simulink model "receive"  (R2024b)
settings: Solver=FixedStepAuto  StartTime=0.0  StopTime=10.0  RelTol=1e-3
settings Model: Creator=Amin  LastModifiedBy=Amin
settings OptimizationCC: DefaultParameterBehavior=Inlined  EnhancedBackFolding=on  PassReuseOutputArgsAs=Individual arguments  ZeroExternalMemoryAtStartup=off  ZeroInternalMemoryAtStartup=off  OptimizeBlockOrder=speed  DifferentSizesBufferReuse=on  OptimizationCustomize=off  EfficientTunableParamExpr=on
settings DebuggingCC: ParameterTunabilityLossMsg=error
settings SFSimCC: MATLABDynamicMemAlloc=off
settings RTWCC: Description=Embedded Coder  SystemTargetFile=ert.tlc  GenCodeOnly=on  TemplateMakefile=ert_default_tmf  DataTypeReplacement=CDataTypesFixedWidth  TargetLang=C++
settings CodeAppCC: ForceParamTrailComments=on  IgnoreCustomStorageClasses=off  OperatorAnnotations=on  SimulinkDataObjDesc=on  SFDataObjDesc=on  InsertBlockDesc=on
settings ERTTargetCC: TargetLangStandard=C++11 (ISO)  GenerateSampleERTMain=on  SupportAbsoluteTime=off  CodeInterfacePackaging=C++ class  SupportNonFinite=off  SupportComplex=off  RootIOFormat=Structure reference  ERTCustomFileTemplate=example_file_process.tlc  ERTFilePackagingFormat=Compact  MaxIdInt64=INT64_MAX  MinIdInt64=INT64_MIN  MaxIdUint64=UINT64_MAX  MaxIdInt32=INT32_MAX  MinIdInt32=INT32_MIN  MaxIdUint32=UINT32_MAX  MaxIdInt16=INT16_MAX  MinIdInt16=INT16_MIN  MaxIdUint16=UINT16_MAX  MaxIdInt8=INT8_MAX  MinIdInt8=INT8_MIN  MaxIdUint8=UINT8_MAX

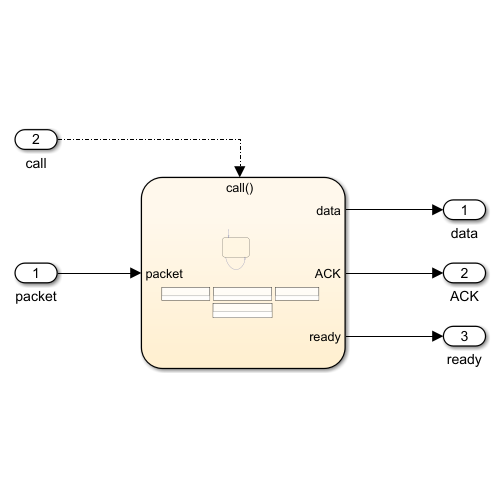
[thumbnail: Simulink's stored preview of the top-level diagram]
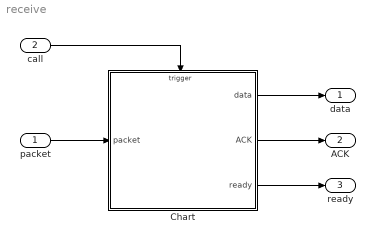
== system receive ==
  packet : Inport
  call : Inport  Port=2  OutputFunctionCall=on
  Chart : Stateflow chart  TreatAsAtomicUnit=on
  data : Outport
  ACK : Outport  Port=2
  ready : Outport  Port=3  OutDataTypeStr=boolean
  wires:
  packet/1 -> Chart/1(packet)
  Chart/1(data) -> data/1
  Chart/2(ACK) -> ACK/1
  call/1 -> Chart/Trigger
  Chart/3(ready) -> ready/1

== stateflow chart receive/Chart ==
  settings: executeAtInitialization=1
  state state
  (default) -> state
  state -> state : [call && check_packet(packet, tag)]{[data, ACK, c_ack] = send_data_ack(packet, c_ack); tag = 1-tag; send(ready);}
  data: f function_output; p function_input; t function_input; value function_input; crc_tag function_input; header function_output; polynomial function_input; p function_input; d function_output; a function_output; c function_input; nc function_output; value function_input; header function_output; polynomial function_input; data output uint8 =0; packet input uint16; ACK output uint8 =0; c_ack local uint8 =0; tag local single =1
  events: call input FUNCTION_CALL_EVENT; ready output EITHER_EDGE_EVENT
  function f = check_packet(p, t):
    | function f = check_packet(p, t)
    | 
    |     header = uint8(bitshift(p, -9));
    |     raw_data = uint8(bitand(p, 0x00FF));
    |     checktag = bitget(p, 9);
    |     if crc4(raw_data, tag, 19) == header && checktag == t
    |         f = true;
    |     else
    |         f = false;
    |     end
    |     
    | end
  function header = crc4(value, crc_tag, polynomial):
    | function header = crc4(value, crc_tag, polynomial)
    |         
    |     % Initialize the CRC register to 0
    |     crc = uint16(0);
    |     input = bitor(uint16(value), bitshift(uint16(crc_tag), 8));
    |         
    |     % Loop over each bit in the input byte (MSB first)
    |     for i = 8:-1:-4
    |         % XOR the MSB of the input with the MSB of the CRC register
    |         crc = bitxor(crc, bitand(bitshift(input, -i), 1));  % Shift input and XOR
    |             
    |         % If the MSB of the CRC is 1, perform the polynomial division (XOR)
    |         if bitget(crc, 5)  % Check if MSB (bit 5) of 8-bit crc is set
    |            crc = bitxor(crc, polynomial);  % Perform division by XOR with polynomial
    |         end
    |             
    |         if i ~= -4
    |             % Shift CRC register left by 1 bit
    |             crc = bitshift(crc, 1);
    |         end
    |     end
    |         
    |     
    |     % Final CRC value is the remainder in the lowest 4 bits
    |     header = uint8(bitand(crc, 15));  % Mask to get the lower 4 bits as the CRC result
    | end
  function [d, a, nc]= send_data_ack(p, c):
    | function [d, a, nc]= send_data_ack(p, c)
    | 
    |     d = uint8(bitand(p, 0x00FF));
    | 
    |     a = bitor(uint8(c), bitshift(uint8(ack_crc(uint8(c), 19)), 4));
    | 
    |     if c == 15
    |         nc = uint8(0);
    |     else
    |         nc = uint8(c+1);
    |     end
    | 
    | end
  function header = ack_crc(value, polynomial):
    | function header = ack_crc(value, polynomial)
    |         
    |     % Initialize the CRC register to 0
    |     crc = uint8(0);
    |         
    |     % Loop over each bit in the input byte (MSB first)
    |     for i = 7:-1:-4
    |         % XOR the MSB of the input with the MSB of the CRC register
    |         crc = bitxor(crc, bitand(bitshift(value, -i), 1));  % Shift input and XOR
    |             
    |         % If the MSB of the CRC is 1, perform the polynomial division (XOR)
    |         if bitget(crc, 5)  % Check if MSB (bit 5) of 8-bit crc is set
    |            crc = bitxor(crc, polynomial);  % Perform division by XOR with polynomial
    |         end
    |             
    |         if i ~= -4
    |             % Shift CRC register left by 1 bit
    |             crc = bitshift(crc, 1);
    |         end
    |     end
    |         
    |     
    |     % Final CRC value is the remainder in the lowest 4 bits
    |     header = bitand(crc, 15);  % Mask to get the lower 4 bits as the CRC result
    | end
